simulink model "Modelisation_4_MDI_sans_arbre_telescopique"  (R2015a)
settings: Solver=ode45  StartTime=0.0  StopTime=3  MaxStep=0.001  RelTol=1e-3
values from neighbouring files (symbols this model uses):
  s = tf('s')    [A_3_LoopShaping.m]    (also in A_4_Hinfini.m = zpk('s'))
  X = [0;0;0;0;0;0;0;0]    [A_1_Data.m]
  Y = [0;0;0;0;0;0;0;0]    [A_1_Data.m]
undefined symbols (not defined in the file or in its folder): sfun3d, Z
libraries: sm_lib x280, nesl_utility x10
(part 9 of 9)

== matlab function Modelisation_4_MDI_sans_arbre_telescopique/MDI_Clavel/Clavel ==
  data: d2P input; alpha input; dalpha input; d2alpha input; Jinv input; T output
function T = fcn(d2P,alpha,dalpha,d2alpha,Jinv)



alpha1=alpha(1) ;alpha2=alpha(2) ; alpha3=alpha(3) ;
dalpha1=dalpha(1) ;dalpha2=dalpha(2) ; dalpha3=dalpha(3) ;
d2alpha1=d2alpha(1) ;d2alpha2=d2alpha(2) ; d2alpha3=d2alpha(3) ;

%% les constantes
    l1 = 0.19992; 
    phi2 = 2*pi/3;
    phi3 = 4*pi/3;

 % Constantes mecaniques
 IA=0.0067 ;
 mA=0.07604 ;
 mC = 0.00564 ; 
 mB =2*0.01438 ;
 mN = 0.04157 ;
 g=[0;0;-9.98 ] ;
    
% Fin

%%  accelerations des points Ci :
% dOCi : la derivee partielle de OCi par rapport au alphai
% d2OCi : la deuxieme derivee partielle de OCi par rapport au alphai

dOC1_1=[-l1*sin(alpha1) ; 0 ; -l1*cos(alpha1)] ; 
dOC2_2=[-l1*sin(alpha2)*cos(phi2) ; -l1*sin(alpha2)*sin(phi2) ; -l1*cos(alpha2)] ;
dOC3_3=[-l1*sin(alpha3)*cos(phi3) ; -l1*sin(alpha3)*sin(phi3) ; -l1*cos(alpha3)] ;

d2OC1_1=[-l1*cos(alpha1) ; 0 ; l1*sin(alpha1)] ;
d2OC2_2=[-l1*cos(alpha2)*cos(phi2) ; -l1*cos(alpha2)*sin(phi2) ; l1*sin(alpha2)] ;
d2OC3_3=[-l1*cos(alpha3)*cos(phi3) ; -l1*cos(alpha3)*sin(phi3) ; l1*sin(alpha3)] ;

d2OC1 = d2OC1_1*dalpha1^2 + dOC1_1*d2alpha1;
d2OC2 = d2OC2_2*dalpha2^2 + dOC2_2*d2alpha2;
d2OC3 = d2OC3_3*dalpha3^2 + dOC3_3*d2alpha3;
%Fin

                                                   %% Modele dynamique etabli par Clavel:
%% Le couple C1_ :
 C1_=dOC1_1'*( ( (mA+mB)/3+mC+IA/l1^2 )*d2OC1 +mB/6*d2P -(mC+(mA+mB)/2)*g ) + (Jinv*[1;0;0])'*(  (mN+mB)*d2P +mB/6*(d2OC1+d2OC2+d2OC3)-(mN+3*mB/2)*g ) ;
  C2_=dOC2_2'*( ( (mA+mB)/3+mC+IA/l1^2 )*d2OC2 +mB/6*d2P -(mC+(mA+mB)/2)*g ) + (Jinv*[0;1;0])'*(  (mN+mB)*d2P +mB/6*(d2OC1+d2OC2+d2OC3)-(mN+3*mB/2)*g ) ;
 C3_=dOC3_3'*( ( (mA+mB)/3+mC+IA/l1^2 )*d2OC3 +mB/6*d2P -(mC+(mA+mB)/2)*g ) + (Jinv*[0;0;1])'*(  (mN+mB)*d2P +mB/6*(d2OC1+d2OC2+d2OC3)-(mN+3*mB/2)*g ) ;

 T1=C1_/12  ;
 T2=C2_/12  ;
 T3=C3_/12  ;
 T=[T1;T2;T3];

== matlab function Modelisation_4_MDI_sans_arbre_telescopique/MDI_Clavel/J_invrsee ==
  data: P0 input; Jinv output
function Jinv = Jinv(P0)

   %% les constantes
    l1 = 0.19992; 
    l2 = 0.334; 
    r = 0.126; 
    phi2 = 2*pi/3;
    phi3 = 4*pi/3;

%% projection de P sur Ri
A2=[cos(phi2) sin(phi2) 0
    -sin(phi2) cos(phi2) 0
    0            0      1 ]; 
A3=[cos(phi3) sin(phi3) 0
    -sin(phi3) cos(phi3) 0
    0            0      1 ];
p2=A2*P0; p3=A3*P0 ;

x1=P0(1); y1=P0(2) ; z1=P0(3) ; %% p1=p
x2=p2(1); y2=p2(2) ; z2=p2(3) ;
x3=p3(1); y3=p3(2) ; z3=p3(3) ;

%% Calcule de ABi et ei :
AB1=sqrt(z1^2+(x1-r)^2);
e1=sqrt(l2^2-y1^2); 
AB2=sqrt(z2^2+(x2-r)^2);
e2=sqrt(l2^2-y2^2);
AB3=sqrt(z3^2+(x3-r)^2);
e3=sqrt(l2^2-y3^2);

%% calcul de alpha1
gama1=acos((AB1^2 + l1^2 - e1^2)/(2*l1*AB1));
gama2=acos((AB2^2 + l1^2 - e2^2)/(2*l1*AB2));
gama3=acos((AB3^2 + l1^2 - e3^2)/(2*l1*AB3));

%% =========== Calcule de  J1  ================
% J1 est defini par : dalpha1= J1*dP
AB1 = sqrt(z1^2+(x1-r)^2);
AH1 = AB1-l1*cos(gama1);
D1=l1*AB1*sin(gama1) ;
a1 = AH1*(x1-r)/AB1/D1 +  z1/( z1^2 + (x1-r)^2 );
a2 = y1/D1 ;
a3 = AH1*z1/AB1/D1 -(x1-r)/( z1^2 + (x1-r)^2 ) ;
j1= [a1 a2 a3] ;

%% =========== Calcule de  J2  ================
% J2 est defini par : dalpha2 = J2*A2*dP
AB2 = sqrt(z2^2+(x2-r)^2);
AH2 = AB2-l1*cos(gama2);
D2=l1*AB2*sin(gama2) ;
a4 = AH2*(x2-r)/AB2/D2 + z2/( z2^2 + (x2-r)^2 ) ;
a5 = y2/D2;
a6 = AH2*z2/AB2/D2 -(x2-r)/( z2^2 + (x2-r)^2 );
j2=[a4 a5 a6]*A2;

%%  ========= (dAlpha3)  ================

AB3 = sqrt(z3^2+(x3-r)^2) ;
AH3 = AB3-l1*cos(gama3) ;
D3=l1*AB3*sin(gama3) ;
a7 = AH3*(x3-r)/AB3/D3 + z3/( z3^2 + (x3-r)^2 ) ;
a8 = y3/D3 ;
a9 = AH3*z3/AB3/D3 -(x3-r)/( z3^2 + (x3-r)^2 ) ;
j3=[ a7 a8 a9]*A3 ;

%% La matrice inverse de J
Jinv=inv([ j1 ; j2 ; j3 ]) ;

== matlab function Modelisation_4_MDI_sans_arbre_telescopique/Trajectoir1 ==
  data: ne input; P output; dP output; d2P output; t input
function [P,dP,d2P]= fcn(ne,t)

%% Menu
% 1 ==> Ligne horizontal
% 2==>  Ligne suivant l'axe oz
% 3==> Cercle
% 4==> Ligne x=y
 z0=-0.08789  ; zpi=-0.3;
B= (z0+zpi)/2 ; A= (z0-zpi)/2 ; 
f = 9; f2 = 5 ;
R=0.2;
%% vers le Plan Z=-0.3
if (t<pi/f && (ne == 1 || ne == 3 ||  ne == 0 || ne == 4 || ne == 5 ||  ne == 6))
n= 2 ; 
elseif( (ne == 4 || ne == 5 ||  ne == 6)  &&  (t<3*pi/2/f) ) % vers le point (0 , R , -0.3)
n=1 ;
else
n =ne ;
end

%% le trajecoir
switch n
    
    case 0
        
        % La position
        x = R*sin(f*t)  ; y=0 ;
        z=  zpi ;
        P = [ x ; y ; z ];
        % La vitess
        dx = f*R*cos(f*t)  ; dy=0 ;
        dz= 0 ;
        dP = [ dx ; dy ; dz ];
        % L'acceleration :
        d2x = -f^2*R*sin(f*t) ; d2y=0 ;
        d2z =  0;
        d2P = [ d2x ; d2y ; d2z ];
        % L'a _coup :
        d3x = -f^3*R*cos(f*t) ; d3y=0 ;
        d3z =  0;
        d3P = [ d3x ; d3y ; d3z ];
    case 1   
        % La position
        y = R*sin(f*t)  ; x=0 ;
        z= zpi  ;
        P = [ x ; y ; z ];
        % La vitess
        dy = f*R*cos(f*t)  ; dx=0 ;
        dz= 0 ;
        dP = [ dx ; dy ; dz ];
        % L'acceleration :
        d2y = -f^2*R*sin(f*t) ; d2x=0 ;
        d2z =  0;
        d2P = [ d2x ; d2y ; d2z ];
        % L'a _coup :
        d3y = -f^3*R*cos(f*t) ; d3x=0 ;
        d3z =  0;
        d3P = [ d3x ; d3y ; d3z ];
    case 2
        % La position 
        x = 0 ; y=0 ;
        z= A*cos(f*t) + B ; 
        P = [ x ; y ; z ];
        % La vitess
        dx = 0 ; dy=0 ;
        dz= -f*A*sin(f*t) ;
        dP = [ dx ; dy ; dz ];
        % L'acceleration :
        d2x = 0 ; d2y=0 ;
        d2z = -f^2*A*cos(f*t) ;
        d2P = [ d2x ; d2y ; d2z ];
        % L a_coup (jerk) :
        d3x = 0 ; d3y=0 ;
        d3z = f^3*A*sin(f*t) ;
        d3P = [ d3x ; d3y ; d3z ];
        
        %%
    case 3
        R=0.12;
        y = R*sin(f*t)  ; x=2*y;
        z= zpi  ;
        P = [ x ; y ; z ];
        % La vitess
        dy = f*R*cos(f*t)  ; dx=2*dy ;
        dz= 0 ;
        dP = [ dx ; dy ; dz ];
        % L'acceleration :
        d2y = -f^2*R*sin(f*t) ; d2x=2*d2y ;
        d2z =  0;
        d2P = [ d2x ; d2y ; d2z ];
        % L'a _coup :
        d3y = -f^3*R*cos(f*t) ; d3x=2*d3y ;
        d3z =  0;
        d3P = [ d3x ; d3y ; d3z ];
    case 4 % Cerecl XY
        x=R*cos(f*t) ; y=R*sin(f*t) ; z=zpi  ;
        dx=-f*R*sin(f*t) ; dy=f*R*cos(f*t)  ;  dz=0;
        d2x=-f^2*R*cos(f*t) ; d2y=-f^2*R*sin(f*t)  ;  d2z=0;
        P=[x ; y ; z];
        dP=[dx ; dy ; dz];
        d2P=[d2x ; d2y ; d2z];
        % L'a _coup :
        d3x=f^3*R*sin(f*t) ; d3y=-f^3*R*cos(f*t)  ;  d3z=0;
        d3P=[d3x ; d3y ; d3z];
        
    case 5 % ZY   
        x=0 ; y=R*sin(f*t) ; z=0.5*R*cos(f*t) + zpi  ;
        dx=0 ; dy=f*R*cos(f*t)  ;  dz=-f*R*sin(f*t);
        d2x=0 ; d2y=-f^2*R*sin(f*t)  ;  d2z=-f^2*R*cos(f*t);
        P=[x ; y ; z];
        dP=[dx ; dy ; dz];
        d2P=[d2x ; d2y ; d2z];
        d3x=0 ; d3y=-f^3*R*cos(f*t)  ;  d3z=f^3*R*sin(f*t);
        d3P=[d3x ; d3y ; d3z];
%     case 6 %Cercle ZX
%         y=0 ; x=R*sin(f*t) ; z=R*cos(f*t) +zpi;
%         dy=0 ; dx=f*R*cos(f*t)  ;  dz=-f*R*sin(f*t);
%         d2y=0 ; d2x=-f^2*R*sin(f*t)  ;  d2z=-f^2*R*cos(f*t);
%         d3y=0 ; d3x=-f^3*R*cos(f*t)  ;  d3z=f^3*R*sin(f*t);
%         P=[x ; y ; z];
%         dP=[dx ; dy ; dz];
%         d2P=[d2x ; d2y ; d2z];
%         d3P = [ d3x ; d3y ; d3z ];
%     case 7  % Les derivees sont a corriger
%         R=0.00*sin(f2*t) ; A=0.1270 ;
%         x=R*cos(f*t) ; y=R*sin(f*t) ;
%         z= A*sin(f2*t) -0.2 ;
%         dx=-f*R*sin(f*t) ; dy=f*R*cos(f*t)  ;  
%         dz= f2*A*cos(f2*t) ;
%         d2x=-f^2*R*cos(f*t) ; d2y=-f^2*R*sin(f*t)  ;
%         d2z = -f2^2*A*sin(f2*t) ;
%         P=[x ; y ; z];
%         dP=[dx ; dy ; dz];
%         d2P=[d2x ; d2y ; d2z];
%         % L'a _coup :
%         d3x=f^3*R*sin(f*t) ; d3y=-f^3*R*cos(f*t)  ;
%         d3z = -f2^3*A*cos(f2*t) ;
%         d3P=[d3x ; d3y ; d3z];
    case 8
        x=0 ; y=0 ; z=z0 ;
        P=[x ; y ; z];
        dP=[0 ; 0 ; 0];
        d2P=[0 ; 0 ; 0];
        d3P=[0 ; 0 ; 0];
        
    otherwise
        P=[0 ; 0 ; 0];
        dP=[0 ; 0 ; 0];
        d2P=[0 ; 0 ; 0];
        d3P = [ 0 ; 0 ; 0 ];
end
